simulink model "tests"  (R2024b)
settings: Solver=VariableStepAuto  StartTime=0.0  StopTime=1  RelTol=1e-3  AbsTol=1e-3  EnableMultiTasking=on
values from neighbouring files (symbols this model uses):
  m = obj.Br *obj.volume / obj.mu    [External_Magnet2.m]
  N = gridSizes(k)    [Test.m]
  Params = Sim_Param_Setup    [Sim_Open.m]
undefined symbols (not defined in the file or in its folder): X, Y, Z
libraries: sm_lib x88, vrlib x72, nesl_utility x52, matrix_library x46, sharedtransform x6
(part 3 of 5)

== system tests/Subsystem/Single_Arm/Plate_2/Torques and Forces ==
  m_slave : Inport
  Pos_Slave : Inport  Port=2
  M1 : Inport  Port=3
  Pos_Plate1 : Inport  Port=4
  M3 : Inport  Port=5
  Pos_Plate3 : Inport  Port=6
  M4 : Inport  Port=7
  Pos_Plate4 : Inport  Port=8
  M5 : Inport  Port=9
  Pos_Plate5 : Inport  Port=10
  M6 : Inport  Port=11
  Pos_Plate6 : Inport  Port=12
  Add{,1..4} (5 alike) : Sum  Inputs=+-
  Magnetic Forces : Subsystem
  Magnetic Torques : Subsystem
      settings: PortSchema="{\"entries\":[{\"content\":{\"sides\":[{\"content\":{\"connectorIds\":[\"In1\",\"In2\",\"In3\",\"In4\",\"In5\",\"In6\",\"In7\",\"In8\",\"In9\",\"In10\",\"In11\"]},\"type\":\"ConnectorPlacement.EquallySpacedRectSide\",\"uuid\":\"6f05c61b-28f4-4565-bbea-1be0fb93c6f0\"},{\"content\":{\"connectorIds\":[\"Out1\"],\"side\":\"RIGHT\"},\"type\":\"ConnectorPlacement.EquallySpacedRectSide\",\"uuid\":\"8634642c-fc93-4182-aaec-4f6aca47cd70\"},{\"content\":{\"connectorIds\":[\"LConn1\"],\"side\":\"TOP\"},\"type\":\"ConnectorPlacement.EquallySpacedRectSide\",\"uuid\":\"4c29c46f-a8de-4915-ac6e-9828579e7b84\"}]},\"type\":\"ConnectorPlacement.EquallySpacedConnector\",\"uuid\":\"3da81916-5d74-4352-a0fa-851a5433a86b\"}],\"packageUris\":[\"http://schema.mathworks.com/mf0/Connector/R2020b\"],\"version\":\"1.0\"}"
  brick reference : PMIOPort  Side=Left
  Forces : Outport
  Torques : Outport  Port=2
  wires:
  m_slave/1 -> Magnetic Forces/1(m_slave), Magnetic Torques/1(m_slave)
  Pos_Slave/1 -> Add4/1, Add3/1, Add2/1, Add1/1, Add/1
  Pos_Plate1/1 -> Add/2
  M1/1 -> Magnetic Torques/2(M1), Magnetic Forces/2(M1)
  Add/1 -> Magnetic Torques/7(r1), Magnetic Forces/7(r1)
  Pos_Plate6/1 -> Add4/2
  Pos_Plate5/1 -> Add3/2
  Pos_Plate4/1 -> Add2/2
  Pos_Plate3/1 -> Add1/2
  M3/1 -> Magnetic Forces/3(M3), Magnetic Torques/3(M3)
  Add1/1 -> Magnetic Torques/8(r3), Magnetic Forces/8(r3)
  M4/1 -> Magnetic Forces/4(M4), Magnetic Torques/4(M4)
  M5/1 -> Magnetic Forces/5(M5), Magnetic Torques/5(M5)
  M6/1 -> Magnetic Forces/6(M6), Magnetic Torques/6(M6)
  Add2/1 -> Magnetic Forces/9(r4), Magnetic Torques/9(r4)
  Add3/1 -> Magnetic Forces/10(r5), Magnetic Torques/10(r5)
  Add4/1 -> Magnetic Forces/11(r6), Magnetic Torques/11(r6)
  Magnetic Forces/1(Forces) -> Forces/1
  Magnetic Torques/1(Torque) -> Torques/1
  connections:
  brick reference/RConn1 -- Magnetic Torques/LConn1

== system tests/Subsystem/Single_Arm/Plate_3/Subsystem ==
  Slave_Moment : Inport
  Slave_Pos : Inport  Port=2
  Source_Moment : Inport  Port=3
  Source_Pos : Inport  Port=4
  Add : Sum  Inputs=+-
  Add1 : Sum  Inputs=+-
  Add2 : Sum  Inputs=+-
  Add3 : Sum  Inputs=+++
  Constant : Constant  Value=-3
  Constant1 : Constant  Value=-4
  Cross Product : matrix_library/Cross Product
  Dot Product : DotProduct  OutDataTypeStr=Inherit: Inherit via internal rule
  Dot Product1 : DotProduct  OutDataTypeStr=Inherit: Inherit via internal rule
  Gain : Gain  Gain=4*pi*1e-7/(4*pi)
  Gain1 : Gain  Gain=3
  Gain2 : Gain  Gain=3*4*pi*1e-7/(4*pi)
  Gain3 : Gain  Gain=5
  IdentityMatrix : IdentityMatrix  OutputDimensions=3
  Matrix Multiply : Product  Multiplication=Matrix(*)
  Matrix Multiply1 : Product  Multiplication=Matrix(*)
  Normalize Vector : vrlib/Utilities/Normalize Vector  maxzero=0
  Normalize Vector1 : vrlib/Utilities/Normalize Vector  maxzero=0
  Power : Math  Operator=pow
  Power1 : Math  Operator=pow
  Product{,1..5} (6 alike) : Product
  Sqrt : Sqrt
  Sqrt1 : Sqrt
  Transpose : Math  Operator=transpose
  m dot m : DotProduct  OutDataTypeStr=Inherit: Inherit via internal rule
  r dot m_master : DotProduct  OutDataTypeStr=Inherit: Inherit via internal rule
  r dot m_slave : DotProduct  OutDataTypeStr=Inherit: Inherit via internal rule
  Source_Torque : Outport
  Source_Force : Outport  Port=2
  wires:
  Power/1 -> Gain/1
  Transpose/1 -> Matrix Multiply/2
  Gain1/1 -> Add/1
  Matrix Multiply/1 -> Gain1/1
  Sqrt/1 -> Power/1
  Gain/1 -> Product/2
  Dot Product/1 -> Sqrt/1
  Product/1 -> Cross Product/2
  Matrix Multiply1/1 -> Product/1
  Normalize Vector/1 -> Transpose/1, Matrix Multiply/1
  IdentityMatrix/1 -> Add/2
  Constant/1 -> Power/2
  Add/1 -> Matrix Multiply1/1
  Slave_Pos/1 -> Add1/1
  Source_Pos/1 -> Add1/2
  Cross Product/1 -> Source_Torque/1
  Slave_Moment/1 -> Cross Product/1, Product2/2, m dot m/1, r dot m_slave/2
  Normalize Vector1/1 -> r dot m_slave/1, r dot m_master/1, Product4/2
  Add3/1 -> Product5/2
  Gain2/1 -> Product5/1
  Product4/1 -> Add3/3
  Dot Product1/1 -> Sqrt1/1
  Gain3/1 -> Add2/2
  r dot m_master/1 -> Product3/2, Product2/1
  Source_Moment/1 -> Matrix Multiply1/2, m dot m/2, Product1/2, r dot m_master/2
  m dot m/1 -> Add2/1
  Power1/1 -> Gain2/1
  Sqrt1/1 -> Power1/1
  r dot m_slave/1 -> Product1/1, Product3/1
  Product2/1 -> Add3/2
  Constant1/1 -> Power1/2
  Add2/1 -> Product4/1
  Add1/1 -> Normalize Vector1/1, Dot Product1/2, Dot Product1/1, Dot Product/2, Dot Product/1, Normalize Vector/1
  Product3/1 -> Gain3/1
  Product1/1 -> Add3/1
  Product5/1 -> Source_Force/1

== system tests/Subsystem/Single_Arm/Plate_3/Torques and Forces ==
  m_slave : Inport
  Pos_Slave : Inport  Port=2
  M1 : Inport  Port=3
  Pos_Plate1 : Inport  Port=4
  M2 : Inport  Port=5
  Pos_Plate2 : Inport  Port=6
  M4 : Inport  Port=7
  Pos_Plate4 : Inport  Port=8
  M5 : Inport  Port=9
  Pos_Plate5 : Inport  Port=10
  M6 : Inport  Port=11
  Pos_Plate6 : Inport  Port=12
  Add{,1..4} (5 alike) : Sum  Inputs=+-
  Magnetic Forces : Subsystem
  Magnetic Torques : Subsystem
      settings: PortSchema="{\"entries\":[{\"content\":{\"sides\":[{\"content\":{\"connectorIds\":[\"In1\",\"In2\",\"In3\",\"In4\",\"In5\",\"In6\",\"In7\",\"In8\",\"In9\",\"In10\",\"In11\"]},\"type\":\"ConnectorPlacement.EquallySpacedRectSide\",\"uuid\":\"05771496-45a2-4580-b6ab-cadf9064ee26\"},{\"content\":{\"connectorIds\":[\"Out1\"],\"side\":\"RIGHT\"},\"type\":\"ConnectorPlacement.EquallySpacedRectSide\",\"uuid\":\"b79900f2-9f02-4790-af3a-0fbba66daa11\"},{\"content\":{\"connectorIds\":[\"LConn1\"],\"side\":\"TOP\"},\"type\":\"ConnectorPlacement.EquallySpacedRectSide\",\"uuid\":\"95266051-22b3-46d7-add2-de0ce2a92008\"}]},\"type\":\"ConnectorPlacement.EquallySpacedConnector\",\"uuid\":\"2bf1b23d-6512-437d-b945-3c726b6a255c\"}],\"packageUris\":[\"http://schema.mathworks.com/mf0/Connector/R2020b\"],\"version\":\"1.0\"}"
  brick reference : PMIOPort  Side=Left
  Forces : Outport
  Torques : Outport  Port=2
  wires:
  m_slave/1 -> Magnetic Forces/1(m_slave), Magnetic Torques/1(m_slave)
  Pos_Slave/1 -> Add4/1, Add3/1, Add2/1, Add1/1, Add/1
  Pos_Plate1/1 -> Add/2
  M1/1 -> Magnetic Torques/2(M1), Magnetic Forces/2(M1)
  Add/1 -> Magnetic Torques/7(r1), Magnetic Forces/7(r1)
  Pos_Plate6/1 -> Add4/2
  Pos_Plate5/1 -> Add3/2
  Pos_Plate4/1 -> Add2/2
  Pos_Plate2/1 -> Add1/2
  M2/1 -> Magnetic Forces/3(M2), Magnetic Torques/3(M2)
  Add1/1 -> Magnetic Torques/8(r2), Magnetic Forces/8(r2)
  M4/1 -> Magnetic Forces/4(M4), Magnetic Torques/4(M4)
  M5/1 -> Magnetic Forces/5(M5), Magnetic Torques/5(M5)
  M6/1 -> Magnetic Forces/6(M6), Magnetic Torques/6(M6)
  Add2/1 -> Magnetic Forces/9(r4), Magnetic Torques/9(r4)
  Add3/1 -> Magnetic Forces/10(r5), Magnetic Torques/10(r5)
  Add4/1 -> Magnetic Forces/11(r6), Magnetic Torques/11(r6)
  Magnetic Forces/1(Forces) -> Forces/1
  Magnetic Torques/1(Torque) -> Torques/1
  connections:
  brick reference/RConn1 -- Magnetic Torques/LConn1

== system tests/Subsystem/Single_Arm/Plate_4/Subsystem ==
  Slave_Moment : Inport
  Slave_Pos : Inport  Port=2
  Source_Moment : Inport  Port=3
  Source_Pos : Inport  Port=4
  Add : Sum  Inputs=+-
  Add1 : Sum  Inputs=+-
  Add2 : Sum  Inputs=+-
  Add3 : Sum  Inputs=+++
  Constant : Constant  Value=-3
  Constant1 : Constant  Value=-4
  Cross Product : matrix_library/Cross Product
  Dot Product : DotProduct  OutDataTypeStr=Inherit: Inherit via internal rule
  Dot Product1 : DotProduct  OutDataTypeStr=Inherit: Inherit via internal rule
  Gain : Gain  Gain=4*pi*1e-7/(4*pi)
  Gain1 : Gain  Gain=3
  Gain2 : Gain  Gain=3*4*pi*1e-7/(4*pi)
  Gain3 : Gain  Gain=5
  IdentityMatrix : IdentityMatrix  OutputDimensions=3
  Matrix Multiply : Product  Multiplication=Matrix(*)
  Matrix Multiply1 : Product  Multiplication=Matrix(*)
  Normalize Vector : vrlib/Utilities/Normalize Vector  maxzero=0
  Normalize Vector1 : vrlib/Utilities/Normalize Vector  maxzero=0
  Power : Math  Operator=pow
  Power1 : Math  Operator=pow
  Product{,1..5} (6 alike) : Product
  Sqrt : Sqrt
  Sqrt1 : Sqrt
  Transpose : Math  Operator=transpose
  m dot m : DotProduct  OutDataTypeStr=Inherit: Inherit via internal rule
  r dot m_master : DotProduct  OutDataTypeStr=Inherit: Inherit via internal rule
  r dot m_slave : DotProduct  OutDataTypeStr=Inherit: Inherit via internal rule
  Source_Torque : Outport
  Source_Force : Outport  Port=2
  wires:
  Power/1 -> Gain/1
  Transpose/1 -> Matrix Multiply/2
  Gain1/1 -> Add/1
  Matrix Multiply/1 -> Gain1/1
  Sqrt/1 -> Power/1
  Gain/1 -> Product/2
  Dot Product/1 -> Sqrt/1
  Product/1 -> Cross Product/2
  Matrix Multiply1/1 -> Product/1
  Normalize Vector/1 -> Transpose/1, Matrix Multiply/1
  IdentityMatrix/1 -> Add/2
  Constant/1 -> Power/2
  Add/1 -> Matrix Multiply1/1
  Slave_Pos/1 -> Add1/1
  Source_Pos/1 -> Add1/2
  Cross Product/1 -> Source_Torque/1
  Slave_Moment/1 -> Cross Product/1, Product2/2, m dot m/1, r dot m_slave/2
  Normalize Vector1/1 -> r dot m_slave/1, r dot m_master/1, Product4/2
  Add3/1 -> Product5/2
  Gain2/1 -> Product5/1
  Product4/1 -> Add3/3
  Dot Product1/1 -> Sqrt1/1
  Gain3/1 -> Add2/2
  r dot m_master/1 -> Product3/2, Product2/1
  Source_Moment/1 -> Matrix Multiply1/2, m dot m/2, Product1/2, r dot m_master/2
  m dot m/1 -> Add2/1
  Power1/1 -> Gain2/1
  Sqrt1/1 -> Power1/1
  r dot m_slave/1 -> Product1/1, Product3/1
  Product2/1 -> Add3/2
  Constant1/1 -> Power1/2
  Add2/1 -> Product4/1
  Add1/1 -> Normalize Vector1/1, Dot Product1/2, Dot Product1/1, Dot Product/2, Dot Product/1, Normalize Vector/1
  Product3/1 -> Gain3/1
  Product1/1 -> Add3/1
  Product5/1 -> Source_Force/1

== system tests/Subsystem/Single_Arm/Plate_4/Torques and Forces ==
  m_slave : Inport
  Pos_Slave : Inport  Port=2
  M1 : Inport  Port=3
  Pos_Plate1 : Inport  Port=4
  M2 : Inport  Port=5
  Pos_Plate2 : Inport  Port=6
  M3 : Inport  Port=7
  Pos_Plate3 : Inport  Port=8
  M5 : Inport  Port=9
  Pos_Plate5 : Inport  Port=10
  M6 : Inport  Port=11
  Pos_Plate6 : Inport  Port=12
  Add{,1..4} (5 alike) : Sum  Inputs=+-
  Magnetic Forces : Subsystem
  Magnetic Torques : Subsystem
      settings: PortSchema="{\"entries\":[{\"content\":{\"sides\":[{\"content\":{\"connectorIds\":[\"In1\",\"In2\",\"In3\",\"In4\",\"In5\",\"In6\",\"In7\",\"In8\",\"In9\",\"In10\",\"In11\"]},\"type\":\"ConnectorPlacement.EquallySpacedRectSide\",\"uuid\":\"05771496-45a2-4580-b6ab-cadf9064ee26\"},{\"content\":{\"connectorIds\":[\"Out1\"],\"side\":\"RIGHT\"},\"type\":\"ConnectorPlacement.EquallySpacedRectSide\",\"uuid\":\"b79900f2-9f02-4790-af3a-0fbba66daa11\"},{\"content\":{\"connectorIds\":[\"LConn1\"],\"side\":\"TOP\"},\"type\":\"ConnectorPlacement.EquallySpacedRectSide\",\"uuid\":\"95266051-22b3-46d7-add2-de0ce2a92008\"}]},\"type\":\"ConnectorPlacement.EquallySpacedConnector\",\"uuid\":\"2bf1b23d-6512-437d-b945-3c726b6a255c\"}],\"packageUris\":[\"http://schema.mathworks.com/mf0/Connector/R2020b\"],\"version\":\"1.0\"}"
  brick reference : PMIOPort  Side=Left
  Forces : Outport
  Torques : Outport  Port=2
  wires:
  m_slave/1 -> Magnetic Forces/1(m_slave), Magnetic Torques/1(m_slave)
  Pos_Slave/1 -> Add4/1, Add3/1, Add2/1, Add1/1, Add/1
  Pos_Plate1/1 -> Add/2
  M1/1 -> Magnetic Torques/2(M1), Magnetic Forces/2(M1)
  Add/1 -> Magnetic Torques/7(r1), Magnetic Forces/7(r1)
  Pos_Plate6/1 -> Add4/2
  Pos_Plate5/1 -> Add3/2
  Pos_Plate3/1 -> Add2/2
  Pos_Plate2/1 -> Add1/2
  M2/1 -> Magnetic Forces/3(M2), Magnetic Torques/3(M2)
  Add1/1 -> Magnetic Torques/8(r2), Magnetic Forces/8(r2)
  M3/1 -> Magnetic Forces/4(M3), Magnetic Torques/4(M3)
  M5/1 -> Magnetic Forces/5(M5), Magnetic Torques/5(M5)
  M6/1 -> Magnetic Forces/6(M6), Magnetic Torques/6(M6)
  Add2/1 -> Magnetic Forces/9(r3), Magnetic Torques/9(r3)
  Add3/1 -> Magnetic Forces/10(r5), Magnetic Torques/10(r5)
  Add4/1 -> Magnetic Forces/11(r6), Magnetic Torques/11(r6)
  Magnetic Forces/1(Forces) -> Forces/1
  Magnetic Torques/1(Torque) -> Torques/1
  connections:
  brick reference/RConn1 -- Magnetic Torques/LConn1

== system tests/Subsystem/Single_Arm/Plate_5/Subsystem ==
  Slave_Moment : Inport
  Slave_Pos : Inport  Port=2
  Source_Moment : Inport  Port=3
  Source_Pos : Inport  Port=4
  Add : Sum  Inputs=+-
  Add1 : Sum  Inputs=+-
  Add2 : Sum  Inputs=+-
  Add3 : Sum  Inputs=+++
  Constant : Constant  Value=-3
  Constant1 : Constant  Value=-4
  Cross Product : matrix_library/Cross Product
  Dot Product : DotProduct  OutDataTypeStr=Inherit: Inherit via internal rule
  Dot Product1 : DotProduct  OutDataTypeStr=Inherit: Inherit via internal rule
  Gain : Gain  Gain=4*pi*1e-7/(4*pi)
  Gain1 : Gain  Gain=3
  Gain2 : Gain  Gain=3*4*pi*1e-7/(4*pi)
  Gain3 : Gain  Gain=5
  IdentityMatrix : IdentityMatrix  OutputDimensions=3
  Matrix Multiply : Product  Multiplication=Matrix(*)
  Matrix Multiply1 : Product  Multiplication=Matrix(*)
  Normalize Vector : vrlib/Utilities/Normalize Vector  maxzero=0
  Normalize Vector1 : vrlib/Utilities/Normalize Vector  maxzero=0
  Power : Math  Operator=pow
  Power1 : Math  Operator=pow
  Product{,1..5} (6 alike) : Product
  Sqrt : Sqrt
  Sqrt1 : Sqrt
  Transpose : Math  Operator=transpose
  m dot m : DotProduct  OutDataTypeStr=Inherit: Inherit via internal rule
  r dot m_master : DotProduct  OutDataTypeStr=Inherit: Inherit via internal rule
  r dot m_slave : DotProduct  OutDataTypeStr=Inherit: Inherit via internal rule
  Source_Torque : Outport
  Source_Force : Outport  Port=2
  wires:
  Power/1 -> Gain/1
  Transpose/1 -> Matrix Multiply/2
  Gain1/1 -> Add/1
  Matrix Multiply/1 -> Gain1/1
  Sqrt/1 -> Power/1
  Gain/1 -> Product/2
  Dot Product/1 -> Sqrt/1
  Product/1 -> Cross Product/2
  Matrix Multiply1/1 -> Product/1
  Normalize Vector/1 -> Transpose/1, Matrix Multiply/1
  IdentityMatrix/1 -> Add/2
  Constant/1 -> Power/2
  Add/1 -> Matrix Multiply1/1
  Slave_Pos/1 -> Add1/1
  Source_Pos/1 -> Add1/2
  Cross Product/1 -> Source_Torque/1
  Slave_Moment/1 -> Cross Product/1, Product2/2, m dot m/1, r dot m_slave/2
  Normalize Vector1/1 -> r dot m_slave/1, r dot m_master/1, Product4/2
  Add3/1 -> Product5/2
  Gain2/1 -> Product5/1
  Product4/1 -> Add3/3
  Dot Product1/1 -> Sqrt1/1
  Gain3/1 -> Add2/2
  r dot m_master/1 -> Product3/2, Product2/1
  Source_Moment/1 -> Matrix Multiply1/2, m dot m/2, Product1/2, r dot m_master/2
  m dot m/1 -> Add2/1
  Power1/1 -> Gain2/1
  Sqrt1/1 -> Power1/1
  r dot m_slave/1 -> Product1/1, Product3/1
  Product2/1 -> Add3/2
  Constant1/1 -> Power1/2
  Add2/1 -> Product4/1
  Add1/1 -> Normalize Vector1/1, Dot Product1/2, Dot Product1/1, Dot Product/2, Dot Product/1, Normalize Vector/1
  Product3/1 -> Gain3/1
  Product1/1 -> Add3/1
  Product5/1 -> Source_Force/1

== system tests/Subsystem/Single_Arm/Plate_5/Torques and Forces ==
  m_slave : Inport
  Pos_Slave : Inport  Port=2
  M1 : Inport  Port=3
  Pos_Plate1 : Inport  Port=4
  M2 : Inport  Port=5
  Pos_Plate2 : Inport  Port=6
  M3 : Inport  Port=7
  Pos_Plate3 : Inport  Port=8
  M4 : Inport  Port=9
  Pos_Plate4 : Inport  Port=10
  M6 : Inport  Port=11
  Pos_Plate6 : Inport  Port=12
  Add{,1..4} (5 alike) : Sum  Inputs=+-
  Magnetic Forces : Subsystem
  Magnetic Torques : Subsystem
      settings: PortSchema="{\"entries\":[{\"content\":{\"sides\":[{\"content\":{\"connectorIds\":[\"In1\",\"In2\",\"In3\",\"In4\",\"In5\",\"In6\",\"In7\",\"In8\",\"In9\",\"In10\",\"In11\"]},\"type\":\"ConnectorPlacement.EquallySpacedRectSide\",\"uuid\":\"05771496-45a2-4580-b6ab-cadf9064ee26\"},{\"content\":{\"connectorIds\":[\"Out1\"],\"side\":\"RIGHT\"},\"type\":\"ConnectorPlacement.EquallySpacedRectSide\",\"uuid\":\"b79900f2-9f02-4790-af3a-0fbba66daa11\"},{\"content\":{\"connectorIds\":[\"LConn1\"],\"side\":\"TOP\"},\"type\":\"ConnectorPlacement.EquallySpacedRectSide\",\"uuid\":\"95266051-22b3-46d7-add2-de0ce2a92008\"}]},\"type\":\"ConnectorPlacement.EquallySpacedConnector\",\"uuid\":\"2bf1b23d-6512-437d-b945-3c726b6a255c\"}],\"packageUris\":[\"http://schema.mathworks.com/mf0/Connector/R2020b\"],\"version\":\"1.0\"}"
  brick reference : PMIOPort  Side=Left
  Forces : Outport
  Torques : Outport  Port=2
  wires:
  m_slave/1 -> Magnetic Forces/1(m_slave), Magnetic Torques/1(m_slave)
  Pos_Slave/1 -> Add4/1, Add3/1, Add2/1, Add1/1, Add/1
  Pos_Plate1/1 -> Add/2
  M1/1 -> Magnetic Torques/2(M1), Magnetic Forces/2(M1)
  Add/1 -> Magnetic Torques/7(r1), Magnetic Forces/7(r1)
  Pos_Plate6/1 -> Add4/2
  Pos_Plate4/1 -> Add3/2
  Pos_Plate3/1 -> Add2/2
  Pos_Plate2/1 -> Add1/2
  M2/1 -> Magnetic Forces/3(M2), Magnetic Torques/3(M2)
  Add1/1 -> Magnetic Torques/8(r2), Magnetic Forces/8(r2)
  M3/1 -> Magnetic Forces/4(M3), Magnetic Torques/4(M3)
  M4/1 -> Magnetic Forces/5(M4), Magnetic Torques/5(M4)
  M6/1 -> Magnetic Forces/6(M6), Magnetic Torques/6(M6)
  Add2/1 -> Magnetic Forces/9(r3), Magnetic Torques/9(r3)
  Add3/1 -> Magnetic Forces/10(r4), Magnetic Torques/10(r4)
  Add4/1 -> Magnetic Forces/11(r6), Magnetic Torques/11(r6)
  Magnetic Forces/1(Forces) -> Forces/1
  Magnetic Torques/1(Torque) -> Torques/1
  connections:
  brick reference/RConn1 -- Magnetic Torques/LConn1

== system tests/Subsystem/Single_Arm/Plate_6/Subsystem ==
  Slave_Moment : Inport
  Slave_Pos : Inport  Port=2
  Source_Moment : Inport  Port=3
  Source_Pos : Inport  Port=4
  Add : Sum  Inputs=+-
  Add1 : Sum  Inputs=+-
  Add2 : Sum  Inputs=+-
  Add3 : Sum  Inputs=+++
  Constant : Constant  Value=-3
  Constant1 : Constant  Value=-4
  Cross Product : matrix_library/Cross Product
  Dot Product : DotProduct  OutDataTypeStr=Inherit: Inherit via internal rule
  Dot Product1 : DotProduct  OutDataTypeStr=Inherit: Inherit via internal rule
  Gain : Gain  Gain=4*pi*1e-7/(4*pi)
  Gain1 : Gain  Gain=3
  Gain2 : Gain  Gain=3*4*pi*1e-7/(4*pi)
  Gain3 : Gain  Gain=5
  IdentityMatrix : IdentityMatrix  OutputDimensions=3
  Matrix Multiply : Product  Multiplication=Matrix(*)
  Matrix Multiply1 : Product  Multiplication=Matrix(*)
  Normalize Vector : vrlib/Utilities/Normalize Vector  maxzero=0
  Normalize Vector1 : vrlib/Utilities/Normalize Vector  maxzero=0
  Power : Math  Operator=pow
  Power1 : Math  Operator=pow
  Product{,1..5} (6 alike) : Product
  Sqrt : Sqrt
  Sqrt1 : Sqrt
  Transpose : Math  Operator=transpose
  m dot m : DotProduct  OutDataTypeStr=Inherit: Inherit via internal rule
  r dot m_master : DotProduct  OutDataTypeStr=Inherit: Inherit via internal rule
  r dot m_slave : DotProduct  OutDataTypeStr=Inherit: Inherit via internal rule
  Source_Torque : Outport
  Source_Force : Outport  Port=2
  wires:
  Power/1 -> Gain/1
  Transpose/1 -> Matrix Multiply/2
  Gain1/1 -> Add/1
  Matrix Multiply/1 -> Gain1/1
  Sqrt/1 -> Power/1
  Gain/1 -> Product/2
  Dot Product/1 -> Sqrt/1
  Product/1 -> Cross Product/2
  Matrix Multiply1/1 -> Product/1
  Normalize Vector/1 -> Transpose/1, Matrix Multiply/1
  IdentityMatrix/1 -> Add/2
  Constant/1 -> Power/2
  Add/1 -> Matrix Multiply1/1
  Slave_Pos/1 -> Add1/1
  Source_Pos/1 -> Add1/2
  Cross Product/1 -> Source_Torque/1
  Slave_Moment/1 -> Cross Product/1, Product2/2, m dot m/1, r dot m_slave/2
  Normalize Vector1/1 -> r dot m_slave/1, r dot m_master/1, Product4/2
  Add3/1 -> Product5/2
  Gain2/1 -> Product5/1
  Product4/1 -> Add3/3
  Dot Product1/1 -> Sqrt1/1
  Gain3/1 -> Add2/2
  r dot m_master/1 -> Product3/2, Product2/1
  Source_Moment/1 -> Matrix Multiply1/2, m dot m/2, Product1/2, r dot m_master/2
  m dot m/1 -> Add2/1
  Power1/1 -> Gain2/1
  Sqrt1/1 -> Power1/1
  r dot m_slave/1 -> Product1/1, Product3/1
  Product2/1 -> Add3/2
  Constant1/1 -> Power1/2
  Add2/1 -> Product4/1
  Add1/1 -> Normalize Vector1/1, Dot Product1/2, Dot Product1/1, Dot Product/2, Dot Product/1, Normalize Vector/1
  Product3/1 -> Gain3/1
  Product1/1 -> Add3/1
  Product5/1 -> Source_Force/1

== system tests/Subsystem/Single_Arm/Plate_6/Torques and Forces ==
  m_slave : Inport
  Pos_Slave : Inport  Port=2
  M1 : Inport  Port=3
  Pos_Plate1 : Inport  Port=4
  M2 : Inport  Port=5
  Pos_Plate2 : Inport  Port=6
  M3 : Inport  Port=7
  Pos_Plate3 : Inport  Port=8
  M4 : Inport  Port=9
  Pos_Plate4 : Inport  Port=10
  M5 : Inport  Port=11
  Pos_Plate5 : Inport  Port=12
  Add{,1..4} (5 alike) : Sum  Inputs=+-
  Magnetic Forces : Subsystem
  Magnetic Torques : Subsystem
      settings: PortSchema="{\"entries\":[{\"content\":{\"sides\":[{\"content\":{\"connectorIds\":[\"In1\",\"In2\",\"In3\",\"In4\",\"In5\",\"In6\",\"In7\",\"In8\",\"In9\",\"In10\",\"In11\"]},\"type\":\"ConnectorPlacement.EquallySpacedRectSide\",\"uuid\":\"6f05c61b-28f4-4565-bbea-1be0fb93c6f0\"},{\"content\":{\"connectorIds\":[\"Out1\"],\"side\":\"RIGHT\"},\"type\":\"ConnectorPlacement.EquallySpacedRectSide\",\"uuid\":\"8634642c-fc93-4182-aaec-4f6aca47cd70\"},{\"content\":{\"connectorIds\":[\"LConn1\"],\"side\":\"TOP\"},\"type\":\"ConnectorPlacement.EquallySpacedRectSide\",\"uuid\":\"4c29c46f-a8de-4915-ac6e-9828579e7b84\"}]},\"type\":\"ConnectorPlacement.EquallySpacedConnector\",\"uuid\":\"3da81916-5d74-4352-a0fa-851a5433a86b\"}],\"packageUris\":[\"http://schema.mathworks.com/mf0/Connector/R2020b\"],\"version\":\"1.0\"}"
  Brick reference : PMIOPort  Side=Left
  Forces : Outport
  Torques : Outport  Port=2
  wires:
  m_slave/1 -> Magnetic Forces/1(m_slave), Magnetic Torques/1(m_slave)
  Pos_Slave/1 -> Add4/1, Add3/1, Add2/1, Add1/1, Add/1
  Pos_Plate1/1 -> Add/2
  M1/1 -> Magnetic Torques/2(M1), Magnetic Forces/2(M1)
  Add/1 -> Magnetic Torques/7(r1), Magnetic Forces/7(r1)
  Pos_Plate5/1 -> Add4/2
  Pos_Plate4/1 -> Add3/2
  Pos_Plate3/1 -> Add2/2
  Pos_Plate2/1 -> Add1/2
  M2/1 -> Magnetic Forces/3(M2), Magnetic Torques/3(M2)
  Add1/1 -> Magnetic Torques/8(r2), Magnetic Forces/8(r2)
  M3/1 -> Magnetic Forces/4(M3), Magnetic Torques/4(M3)
  M4/1 -> Magnetic Forces/5(M4), Magnetic Torques/5(M4)
  M5/1 -> Magnetic Forces/6(M5), Magnetic Torques/6(M5)
  Add2/1 -> Magnetic Forces/9(r3), Magnetic Torques/9(r3)
  Add3/1 -> Magnetic Forces/10(r4), Magnetic Torques/10(r4)
  Add4/1 -> Magnetic Forces/11(r5), Magnetic Torques/11(r5)
  Magnetic Forces/1(Forces) -> Forces/1
  Magnetic Torques/1(Torque) -> Torques/1
  connections:
  Brick reference/RConn1 -- Magnetic Torques/LConn1

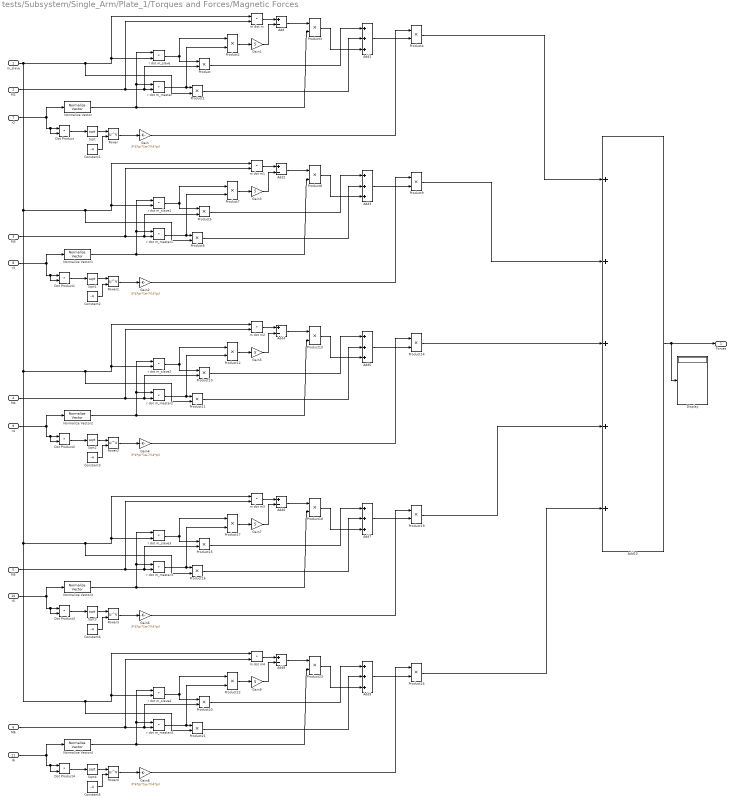
== system tests/Subsystem/Single_Arm/Plate_1/Torques and Forces/Magnetic Forces ==
  m_slave : Inport
  M2 : Inport  Port=2
  M3 : Inport  Port=3
  M4 : Inport  Port=4
  M5 : Inport  Port=5
  M6 : Inport  Port=6
  r2 : Inport  Port=7
  r3 : Inport  Port=8
  r4 : Inport  Port=9
  r5 : Inport  Port=10
  r6 : Inport  Port=11
  Add{,2,4,6,8} (5 alike) : Sum  Inputs=+-
  Add{1,3,5,7,9} (5 alike) : Sum  Inputs=+++
  Add10 : Sum  Inputs=+++++
  Constant{1..5} (5 alike) : Constant  Value=-4
  Display : Display
  Dot Product{,1..4} (5 alike) : DotProduct  OutDataTypeStr=Inherit: Inherit via internal rule
  Gain{,2,4,6,8} (5 alike) : Gain  Gain=3*4*pi*1e-7/(4*pi)
  Gain{1,3,5,7,9} (5 alike) : Gain  Gain=5
  Normalize Vector{,1..4} (5 alike) : vrlib/Utilities/Normalize Vector  maxzero=0
  Power{,1..4} (5 alike) : Math  Operator=pow
  Product{,1..24} (25 alike) : Product
  Sqrt{,1..4} (5 alike) : Sqrt
  m dot m{,1..4} (5 alike) : DotProduct  OutDataTypeStr=Inherit: Inherit via internal rule
  r dot m_master{,1..4} (5 alike) : DotProduct  OutDataTypeStr=Inherit: Inherit via internal rule
  r dot m_slave{,1..4} (5 alike) : DotProduct  OutDataTypeStr=Inherit: Inherit via internal rule
  Forces : Outport
  wires:
  M2/1 -> m dot m/2, Product/2, r dot m_master/2
  r2/1 -> Normalize Vector/1, Dot Product/2, Dot Product/1
  Dot Product/1 -> Sqrt/1
  Sqrt/1 -> Power/1
  Constant1/1 -> Power/2
  Power/1 -> Gain/1
  r dot m_slave/1 -> Product/1, Product2/1
  r dot m_master/1 -> Product2/2, Product1/1
  Product/1 -> Add1/1
  Product1/1 -> Add1/2
  Product2/1 -> Gain1/1
  m dot m/1 -> Add/1
  Gain1/1 -> Add/2
  Normalize Vector/1 -> r dot m_slave/1, r dot m_master/1, Product3/2
  Add/1 -> Product3/1
  Product3/1 -> Add1/3
  Gain/1 -> Product4/1
  Add1/1 -> Product4/2
  Dot Product1/1 -> Sqrt1/1
  Normalize Vector1/1 -> r dot m_slave1/1, r dot m_master1/1, Product8/2
  Product5/1 -> Add3/1
  Add2/1 -> Product8/1
  Gain3/1 -> Add2/2
  m dot m1/1 -> Add2/1
  r dot m_master1/1 -> Product7/2, Product6/1
  Gain2/1 -> Product9/1
  Power1/1 -> Gain2/1
  M3/1 -> m dot m1/2, Product5/2, r dot m_master1/2
  Add3/1 -> Product9/2
  r3/1 -> Dot Product1/2, Dot Product1/1, Normalize Vector1/1
  Sqrt1/1 -> Power1/1
  Product9/1 -> Add10/2
  Product7/1 -> Gain3/1
  Constant2/1 -> Power1/2
  Product8/1 -> Add3/3
  Product6/1 -> Add3/2
  r dot m_slave1/1 -> Product5/1, Product7/1
  Dot Product2/1 -> Sqrt2/1
  Normalize Vector2/1 -> r dot m_slave2/1, r dot m_master2/1, Product13/2
  Product10/1 -> Add5/1
  Add4/1 -> Product13/1
  Gain5/1 -> Add4/2
  m dot m2/1 -> Add4/1
  r dot m_master2/1 -> Product12/2, Product11/1
  Gain4/1 -> Product14/1
  Power2/1 -> Gain4/1
  M4/1 -> m dot m2/2, Product10/2, r dot m_master2/2
  Add5/1 -> Product14/2
  r4/1 -> Normalize Vector2/1, Dot Product2/2, Dot Product2/1
  Sqrt2/1 -> Power2/1
  Product14/1 -> Add10/3
  Product12/1 -> Gain5/1
  Constant3/1 -> Power2/2
  Product13/1 -> Add5/3
  Product11/1 -> Add5/2
  r dot m_slave2/1 -> Product10/1, Product12/1
  Dot Product3/1 -> Sqrt3/1
  Normalize Vector3/1 -> r dot m_slave3/1, r dot m_master3/1, Product18/2
  Product15/1 -> Add7/1
  Add6/1 -> Product18/1
  Gain7/1 -> Add6/2
  m dot m3/1 -> Add6/1
  r dot m_master3/1 -> Product17/2, Product16/1
  Gain6/1 -> Product19/1
  Power3/1 -> Gain6/1
  M5/1 -> m dot m3/2, Product15/2, r dot m_master3/2
  Add7/1 -> Product19/2
  r5/1 -> Dot Product3/2, Dot Product3/1, Normalize Vector3/1
  Sqrt3/1 -> Power3/1
  Product19/1 -> Add10/4
  Product17/1 -> Gain7/1
  Constant4/1 -> Power3/2
  Product18/1 -> Add7/3
  Product16/1 -> Add7/2
  r dot m_slave3/1 -> Product15/1, Product17/1
  Dot Product4/1 -> Sqrt4/1
  Normalize Vector4/1 -> r dot m_slave4/1, r dot m_master4/1, Product23/2
  Product20/1 -> Add9/1
  Add8/1 -> Product23/1
  Gain9/1 -> Add8/2
  m dot m4/1 -> Add8/1
  r dot m_master4/1 -> Product22/2, Product21/1
  Gain8/1 -> Product24/1
  Power4/1 -> Gain8/1
  M6/1 -> m dot m4/2, Product20/2, r dot m_master4/2
  Add9/1 -> Product24/2
  r6/1 -> Normalize Vector4/1, Dot Product4/2, Dot Product4/1
  Sqrt4/1 -> Power4/1
  Product24/1 -> Add10/5
  Product22/1 -> Gain9/1
  Constant5/1 -> Power4/2
  m_slave/1 -> Product21/2, m dot m4/1, r dot m_slave4/2, Product16/2, m dot m3/1, r dot m_slave3/2, Product11/2, m dot m2/1, r dot m_slave2/2, Product6/2, m dot m1/1, r dot m_slave1/2, Product1/2, m dot m/1, r dot m_slave/2
  Product23/1 -> Add9/3
  Product21/1 -> Add9/2
  r dot m_slave4/1 -> Product20/1, Product22/1
  Product4/1 -> Add10/1
  Add10/1 -> Forces/1, Display/1

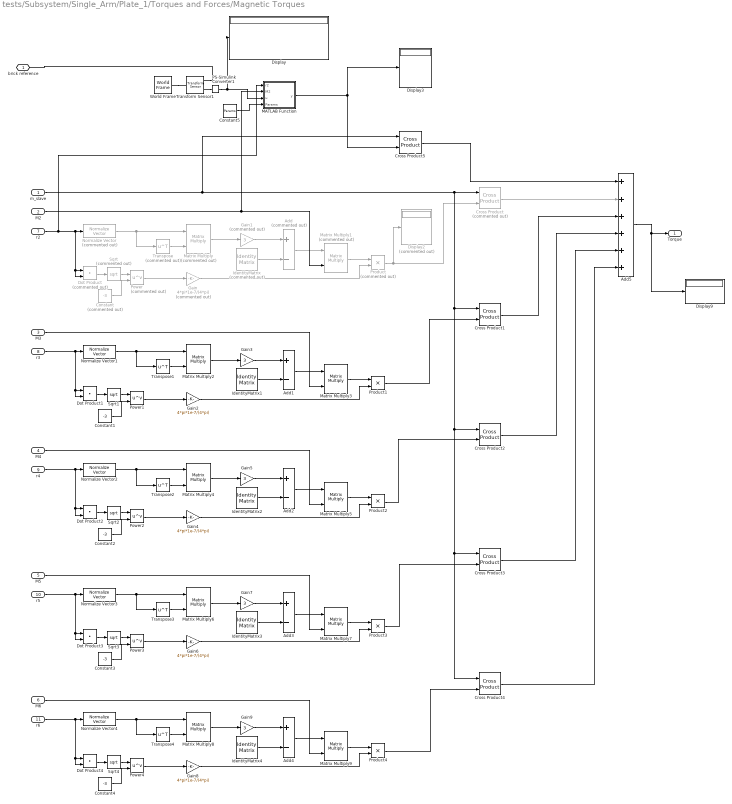
== system tests/Subsystem/Single_Arm/Plate_1/Torques and Forces/Magnetic Torques ==
  m_slave : Inport
  M2 : Inport  Port=2
  M3 : Inport  Port=3
  M4 : Inport  Port=4
  M5 : Inport  Port=5
  M6 : Inport  Port=6
  r2 : Inport  Port=7
  r3 : Inport  Port=8
  r4 : Inport  Port=9
  r5 : Inport  Port=10
  r6 : Inport  Port=11
  Add : Sum  Commented=on  Inputs=+-
  Add{1..4} (4 alike) : Sum  Inputs=+-
  Add5 : Sum  Inputs=++++++
  Constant : Constant  Commented=on  Value=-3
  Constant{1..4} (4 alike) : Constant  Value=-3
  Constant5 : Constant  Value=Params  OutDataTypeStr=Bus:slBus1
  Cross Product : matrix_library/Cross Product  Commented=on
  Cross Product{1..5} (5 alike) : matrix_library/Cross Product
  Display : Display
  Display2 : Display  Commented=on
  Display3 : Display
  Display9 : Display
  Dot Product : DotProduct  Commented=on  OutDataTypeStr=Inherit: Inherit via internal rule
  Dot Product{1..4} (4 alike) : DotProduct  OutDataTypeStr=Inherit: Inherit via internal rule
  Gain : Gain  Commented=on  Gain=4*pi*1e-7/(4*pi)
  Gain1 : Gain  Commented=on  Gain=3
  Gain{2,4,6,8} (4 alike) : Gain  Gain=4*pi*1e-7/(4*pi)
  Gain{3,5,7,9} (4 alike) : Gain  Gain=3
  IdentityMatrix : IdentityMatrix  Commented=on  OutputDimensions=3
  IdentityMatrix{1..4} (4 alike) : IdentityMatrix  OutputDimensions=3
  MATLAB Function : MATLAB Function  TreatAsAtomicUnit=on
  Matrix Multiply : Product  Commented=on  Multiplication=Matrix(*)
  Matrix Multiply1 : Product  Commented=on  Multiplication=Matrix(*)
  Matrix Multiply{2..9} (8 alike) : Product  Multiplication=Matrix(*)
  Normalize Vector : vrlib/Utilities/Normalize Vector  Commented=on  maxzero=0
  Normalize Vector{1..4} (4 alike) : vrlib/Utilities/Normalize Vector  maxzero=0
  PS-Simulink Converter1 : nesl_utility/PS-Simulink Converter  PhysicalDomain=network_engine_domain  SubClassName=ps_output  LeftPortType=input  RightPortType=output  PseudoPeriodic=off  Frequencies=[]  VectorFormat=inherit  Unit=inherit  AffineConversion=off
  Power : Math  Commented=on  Operator=pow
  Power{1..4} (4 alike) : Math  Operator=pow
  Product : Product  Commented=on
  Product{1..4} (4 alike) : Product
  Sqrt : Sqrt  Commented=on
  Sqrt{1..4} (4 alike) : Sqrt
  Transform Sensor1 : sm_lib/Frames and Transforms/Transform Sensor  MeasurementFrame=World  RotationSequence=XYX  SenseAngle=off  SenseAxis=off  SenseQ=off  SenseR=on  SenseRotationSequence=off  SenseOmegaX=off  SenseOmegaY=off  SenseOmegaZ=off  SenseOmega=off  SenseQDot=off  SenseRDot=off  SenseRotationSequenceDot=off  SenseAlphaX=off  SenseAlphaY=off  SenseAlphaZ=off  SenseAlpha=off  SenseQDDot=off  SenseRDDot=off  SenseX=off  SenseY=off  SenseZ=off  SenseXYZ=off  SenseRad=off  SenseAzim=off  SenseDist=off  SenseInc=off  SenseXDot=off  SenseYDot=off  SenseZDot=off  SenseXYZDot=off  SenseRadDot=off  SenseAzimDot=off  SenseDistDot=off  SenseIncDot=off  SenseXDDot=off  SenseYDDot=off  SenseZDDot=off  SenseXYZDDot=off  SenseRadDDot=off  SenseAzimDDot=off  SenseDistDDot=off  SenseIncDDot=off
  Transpose : Math  Commented=on  Operator=transpose
  Transpose{1..4} (4 alike) : Math  Operator=transpose
  World Frame : sm_lib/Frames and Transforms/World Frame
  brick reference : PMIOPort  Side=Left
  Torque : Outport
  wires:
  r2/1 -> MATLAB Function/1(r2), Dot Product/2, Dot Product/1, Normalize Vector/1
  Constant/1 -> Power/2
  Power/1 -> Gain/1
  Normalize Vector/1 -> Transpose/1, Matrix Multiply/1
  Transpose/1 -> Matrix Multiply/2
  Matrix Multiply/1 -> Gain1/1
  IdentityMatrix/1 -> Add/2
  Gain1/1 -> Add/1
  Add/1 -> Matrix Multiply1/1
  M2/1 -> MATLAB Function/2(M2), Matrix Multiply1/2
  Matrix Multiply1/1 -> Product/1
  Gain/1 -> Product/2
  Product/1 -> Cross Product/2, Display2/1
  m_slave/1 -> Cross Product5/1, Cross Product4/1, Cross Product3/1, Cross Product2/1, Cross Product1/1, Cross Product/1
  Dot Product/1 -> Sqrt/1
  Sqrt/1 -> Power/1
  Transpose1/1 -> Matrix Multiply2/2
  Normalize Vector1/1 -> Transpose1/1, Matrix Multiply2/1
  r3/1 -> Dot Product1/2, Dot Product1/1, Normalize Vector1/1
  Matrix Multiply3/1 -> Product1/1
  Matrix Multiply2/1 -> Gain3/1
  IdentityMatrix1/1 -> Add1/2
  Power1/1 -> Gain2/1
  M3/1 -> Matrix Multiply3/2
  Gain3/1 -> Add1/1
  Sqrt1/1 -> Power1/1
  Product1/1 -> Cross Product1/2
  Gain2/1 -> Product1/2
  Add1/1 -> Matrix Multiply3/1
  Dot Product1/1 -> Sqrt1/1
  Constant1/1 -> Power1/2
  Transpose2/1 -> Matrix Multiply4/2
  Normalize Vector2/1 -> Transpose2/1, Matrix Multiply4/1
  r4/1 -> Dot Product2/2, Dot Product2/1, Normalize Vector2/1
  Matrix Multiply5/1 -> Product2/1
  Matrix Multiply4/1 -> Gain5/1
  IdentityMatrix2/1 -> Add2/2
  Power2/1 -> Gain4/1
  M4/1 -> Matrix Multiply5/2
  Gain5/1 -> Add2/1
  Sqrt2/1 -> Power2/1
  Product2/1 -> Cross Product2/2
  Gain4/1 -> Product2/2
  Add2/1 -> Matrix Multiply5/1
  Dot Product2/1 -> Sqrt2/1
  Constant2/1 -> Power2/2
  Transpose3/1 -> Matrix Multiply6/2
  Normalize Vector3/1 -> Transpose3/1, Matrix Multiply6/1
  r5/1 -> Dot Product3/2, Dot Product3/1, Normalize Vector3/1
  Matrix Multiply7/1 -> Product3/1
  Matrix Multiply6/1 -> Gain7/1
  IdentityMatrix3/1 -> Add3/2
  Power3/1 -> Gain6/1
  M5/1 -> Matrix Multiply7/2
  Gain7/1 -> Add3/1
  Sqrt3/1 -> Power3/1
  Product3/1 -> Cross Product3/2
  Gain6/1 -> Product3/2
  Add3/1 -> Matrix Multiply7/1
  Dot Product3/1 -> Sqrt3/1
  Constant3/1 -> Power3/2
  Transpose4/1 -> Matrix Multiply8/2
  Normalize Vector4/1 -> Transpose4/1, Matrix Multiply8/1
  r6/1 -> Dot Product4/2, Dot Product4/1, Normalize Vector4/1
  Matrix Multiply9/1 -> Product4/1
  Matrix Multiply8/1 -> Gain9/1
  IdentityMatrix4/1 -> Add4/2
  Power4/1 -> Gain8/1
  M6/1 -> Matrix Multiply9/2
  Gain9/1 -> Add4/1
  Sqrt4/1 -> Power4/1
  Product4/1 -> Cross Product4/2
  Gain8/1 -> Product4/2
  Add4/1 -> Matrix Multiply9/1
  Dot Product4/1 -> Sqrt4/1
  Constant4/1 -> Power4/2
  Cross Product/1 -> Add5/2
  Cross Product1/1 -> Add5/3
  Cross Product2/1 -> Add5/4
  Cross Product3/1 -> Add5/5
  Cross Product4/1 -> Add5/6
  Add5/1 -> Display9/1, Torque/1
  Constant5/1 -> MATLAB Function/4(Params)
  PS-Simulink Converter1/1 -> Display/1, MATLAB Function/3(u)
  MATLAB Function/1(y) -> Cross Product5/2, Display3/1
  Cross Product5/1 -> Add5/1
  connections:
  Transform Sensor1/RConn1 -- brick reference/RConn1
  Transform Sensor1/RConn2 -- PS-Simulink Converter1/LConn1
  World Frame/RConn1 -- Transform Sensor1/LConn1

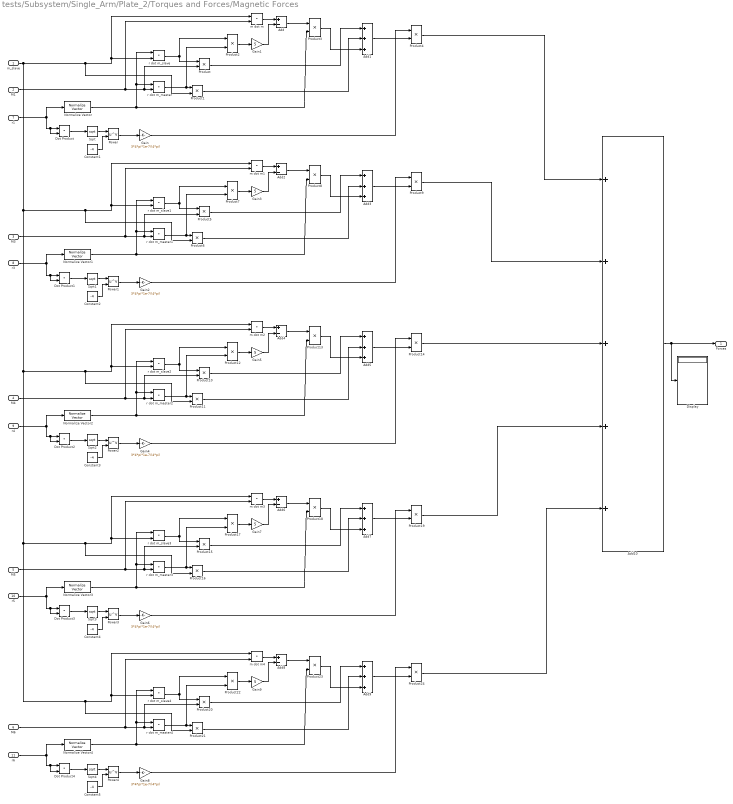
== system tests/Subsystem/Single_Arm/Plate_2/Torques and Forces/Magnetic Forces ==
  m_slave : Inport
  M1 : Inport  Port=2
  M3 : Inport  Port=3
  M4 : Inport  Port=4
  M5 : Inport  Port=5
  M6 : Inport  Port=6
  r1 : Inport  Port=7
  r3 : Inport  Port=8
  r4 : Inport  Port=9
  r5 : Inport  Port=10
  r6 : Inport  Port=11
  Add{,2,4,6,8} (5 alike) : Sum  Inputs=+-
  Add{1,3,5,7,9} (5 alike) : Sum  Inputs=+++
  Add10 : Sum  Inputs=+++++
  Constant{1..5} (5 alike) : Constant  Value=-4
  Display : Display
  Dot Product{,1..4} (5 alike) : DotProduct  OutDataTypeStr=Inherit: Inherit via internal rule
  Gain{,2,4,6,8} (5 alike) : Gain  Gain=3*4*pi*1e-7/(4*pi)
  Gain{1,3,5,7,9} (5 alike) : Gain  Gain=5
  Normalize Vector{,1..4} (5 alike) : vrlib/Utilities/Normalize Vector  maxzero=0
  Power{,1..4} (5 alike) : Math  Operator=pow
  Product{,1..24} (25 alike) : Product
  Sqrt{,1..4} (5 alike) : Sqrt
  m dot m{,1..4} (5 alike) : DotProduct  OutDataTypeStr=Inherit: Inherit via internal rule
  r dot m_master{,1..4} (5 alike) : DotProduct  OutDataTypeStr=Inherit: Inherit via internal rule
  r dot m_slave{,1..4} (5 alike) : DotProduct  OutDataTypeStr=Inherit: Inherit via internal rule
  Forces : Outport
  wires:
  M1/1 -> m dot m/2, Product/2, r dot m_master/2
  r1/1 -> Normalize Vector/1, Dot Product/2, Dot Product/1
  Dot Product/1 -> Sqrt/1
  Sqrt/1 -> Power/1
  Constant1/1 -> Power/2
  Power/1 -> Gain/1
  r dot m_slave/1 -> Product/1, Product2/1
  r dot m_master/1 -> Product2/2, Product1/1
  Product/1 -> Add1/1
  Product1/1 -> Add1/2
  Product2/1 -> Gain1/1
  m dot m/1 -> Add/1
  Gain1/1 -> Add/2
  Normalize Vector/1 -> r dot m_slave/1, r dot m_master/1, Product3/2
  Add/1 -> Product3/1
  Product3/1 -> Add1/3
  Gain/1 -> Product4/1
  Add1/1 -> Product4/2
  Dot Product1/1 -> Sqrt1/1
  Normalize Vector1/1 -> r dot m_slave1/1, r dot m_master1/1, Product8/2
  Product5/1 -> Add3/1
  Add2/1 -> Product8/1
  Gain3/1 -> Add2/2
  m dot m1/1 -> Add2/1
  r dot m_master1/1 -> Product7/2, Product6/1
  Gain2/1 -> Product9/1
  Power1/1 -> Gain2/1
  M3/1 -> m dot m1/2, Product5/2, r dot m_master1/2
  Add3/1 -> Product9/2
  r3/1 -> Dot Product1/2, Dot Product1/1, Normalize Vector1/1
  Sqrt1/1 -> Power1/1
  Product9/1 -> Add10/2
  Product7/1 -> Gain3/1
  Constant2/1 -> Power1/2
  Product8/1 -> Add3/3
  Product6/1 -> Add3/2
  r dot m_slave1/1 -> Product5/1, Product7/1
  Dot Product2/1 -> Sqrt2/1
  Normalize Vector2/1 -> r dot m_slave2/1, r dot m_master2/1, Product13/2
  Product10/1 -> Add5/1
  Add4/1 -> Product13/1
  Gain5/1 -> Add4/2
  m dot m2/1 -> Add4/1
  r dot m_master2/1 -> Product12/2, Product11/1
  Gain4/1 -> Product14/1
  Power2/1 -> Gain4/1
  M4/1 -> m dot m2/2, Product10/2, r dot m_master2/2
  Add5/1 -> Product14/2
  r4/1 -> Normalize Vector2/1, Dot Product2/2, Dot Product2/1
  Sqrt2/1 -> Power2/1
  Product14/1 -> Add10/3
  Product12/1 -> Gain5/1
  Constant3/1 -> Power2/2
  Product13/1 -> Add5/3
  Product11/1 -> Add5/2
  r dot m_slave2/1 -> Product10/1, Product12/1
  Dot Product3/1 -> Sqrt3/1
  Normalize Vector3/1 -> r dot m_slave3/1, r dot m_master3/1, Product18/2
  Product15/1 -> Add7/1
  Add6/1 -> Product18/1
  Gain7/1 -> Add6/2
  m dot m3/1 -> Add6/1
  r dot m_master3/1 -> Product17/2, Product16/1
  Gain6/1 -> Product19/1
  Power3/1 -> Gain6/1
  M5/1 -> m dot m3/2, Product15/2, r dot m_master3/2
  Add7/1 -> Product19/2
  r5/1 -> Dot Product3/2, Dot Product3/1, Normalize Vector3/1
  Sqrt3/1 -> Power3/1
  Product19/1 -> Add10/4
  Product17/1 -> Gain7/1
  Constant4/1 -> Power3/2
  Product18/1 -> Add7/3
  Product16/1 -> Add7/2
  r dot m_slave3/1 -> Product15/1, Product17/1
  Dot Product4/1 -> Sqrt4/1
  Normalize Vector4/1 -> r dot m_slave4/1, r dot m_master4/1, Product23/2
  Product20/1 -> Add9/1
  Add8/1 -> Product23/1
  Gain9/1 -> Add8/2
  m dot m4/1 -> Add8/1
  r dot m_master4/1 -> Product22/2, Product21/1
  Gain8/1 -> Product24/1
  Power4/1 -> Gain8/1
  M6/1 -> m dot m4/2, Product20/2, r dot m_master4/2
  Add9/1 -> Product24/2
  r6/1 -> Normalize Vector4/1, Dot Product4/2, Dot Product4/1
  Sqrt4/1 -> Power4/1
  Product24/1 -> Add10/5
  Product22/1 -> Gain9/1
  Constant5/1 -> Power4/2
  m_slave/1 -> Product21/2, m dot m4/1, r dot m_slave4/2, Product16/2, m dot m3/1, r dot m_slave3/2, Product11/2, m dot m2/1, r dot m_slave2/2, Product6/2, m dot m1/1, r dot m_slave1/2, Product1/2, m dot m/1, r dot m_slave/2
  Product23/1 -> Add9/3
  Product21/1 -> Add9/2
  r dot m_slave4/1 -> Product20/1, Product22/1
  Product4/1 -> Add10/1
  Add10/1 -> Forces/1, Display/1

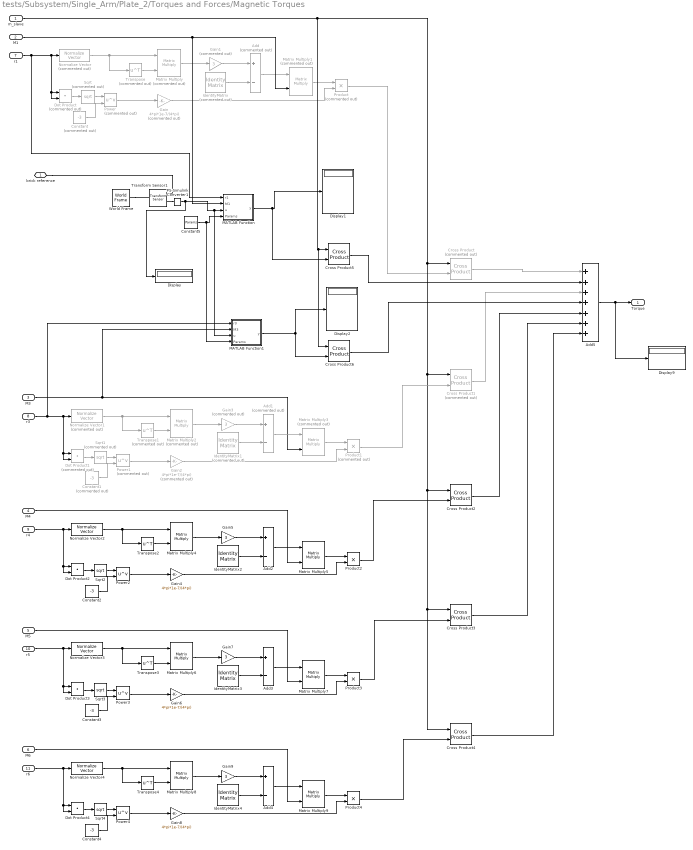
== system tests/Subsystem/Single_Arm/Plate_2/Torques and Forces/Magnetic Torques ==
  m_slave : Inport
  M1 : Inport  Port=2
  M3 : Inport  Port=3
  M4 : Inport  Port=4
  M5 : Inport  Port=5
  M6 : Inport  Port=6
  r1 : Inport  Port=7
  r3 : Inport  Port=8
  r4 : Inport  Port=9
  r5 : Inport  Port=10
  r6 : Inport  Port=11
  Add : Sum  Commented=on  Inputs=+-
  Add1 : Sum  Commented=on  Inputs=+-
  Add2 : Sum  Inputs=+-
  Add3 : Sum  Inputs=+-
  Add4 : Sum  Inputs=+-
  Add5 : Sum  Inputs=+++++++
  Constant : Constant  Commented=on  Value=-3
  Constant1 : Constant  Commented=on  Value=-3
  Constant2 : Constant  Value=-3
  Constant3 : Constant  Value=-3
  Constant4 : Constant  Value=-3
  Constant5 : Constant  Value=Params  OutDataTypeStr=Bus:slBus1
  Cross Product : matrix_library/Cross Product  Commented=on
  Cross Product1 : matrix_library/Cross Product  Commented=on
  Cross Product{2..6} (5 alike) : matrix_library/Cross Product
  Display{,1..2,9} (4 alike) : Display
  Dot Product : DotProduct  Commented=on  OutDataTypeStr=Inherit: Inherit via internal rule
  Dot Product1 : DotProduct  Commented=on  OutDataTypeStr=Inherit: Inherit via internal rule
  Dot Product2 : DotProduct  OutDataTypeStr=Inherit: Inherit via internal rule
  Dot Product3 : DotProduct  OutDataTypeStr=Inherit: Inherit via internal rule
  Dot Product4 : DotProduct  OutDataTypeStr=Inherit: Inherit via internal rule
  Gain : Gain  Commented=on  Gain=4*pi*1e-7/(4*pi)
  Gain1 : Gain  Commented=on  Gain=3
  Gain2 : Gain  Commented=on  Gain=4*pi*1e-7/(4*pi)
  Gain3 : Gain  Commented=on  Gain=3
  Gain4 : Gain  Gain=4*pi*1e-7/(4*pi)
  Gain5 : Gain  Gain=3
  Gain6 : Gain  Gain=4*pi*1e-7/(4*pi)
  Gain7 : Gain  Gain=3
  Gain8 : Gain  Gain=4*pi*1e-7/(4*pi)
  Gain9 : Gain  Gain=3
  IdentityMatrix : IdentityMatrix  Commented=on  OutputDimensions=3
  IdentityMatrix1 : IdentityMatrix  Commented=on  OutputDimensions=3
  IdentityMatrix2 : IdentityMatrix  OutputDimensions=3
  IdentityMatrix3 : IdentityMatrix  OutputDimensions=3
  IdentityMatrix4 : IdentityMatrix  OutputDimensions=3
  MATLAB Function : MATLAB Function  TreatAsAtomicUnit=on
  MATLAB Function1 : MATLAB Function  TreatAsAtomicUnit=on
  Matrix Multiply{,1..3} (4 alike) : Product  Commented=on  Multiplication=Matrix(*)
  Matrix Multiply{4..9} (6 alike) : Product  Multiplication=Matrix(*)
  Normalize Vector : vrlib/Utilities/Normalize Vector  Commented=on  maxzero=0
  Normalize Vector1 : vrlib/Utilities/Normalize Vector  Commented=on  maxzero=0
  Normalize Vector2 : vrlib/Utilities/Normalize Vector  maxzero=0
  Normalize Vector3 : vrlib/Utilities/Normalize Vector  maxzero=0
  Normalize Vector4 : vrlib/Utilities/Normalize Vector  maxzero=0
  PS-Simulink Converter1 : nesl_utility/PS-Simulink Converter  PhysicalDomain=network_engine_domain  SubClassName=ps_output  LeftPortType=input  RightPortType=output  PseudoPeriodic=off  Frequencies=[]  VectorFormat=inherit  Unit=inherit  AffineConversion=off
  Power : Math  Commented=on  Operator=pow
  Power1 : Math  Commented=on  Operator=pow
  Power2 : Math  Operator=pow
  Power3 : Math  Operator=pow
  Power4 : Math  Operator=pow
  Product : Product  Commented=on
  Product1 : Product  Commented=on
  Product2 : Product
  Product3 : Product
  Product4 : Product
  Sqrt : Sqrt  Commented=on
  Sqrt1 : Sqrt  Commented=on
  Sqrt2 : Sqrt
  Sqrt3 : Sqrt
  Sqrt4 : Sqrt
  Transform Sensor1 : sm_lib/Frames and Transforms/Transform Sensor  MeasurementFrame=World  RotationSequence=XYX  SenseAngle=off  SenseAxis=off  SenseQ=off  SenseR=on  SenseRotationSequence=off  SenseOmegaX=off  SenseOmegaY=off  SenseOmegaZ=off  SenseOmega=off  SenseQDot=off  SenseRDot=off  SenseRotationSequenceDot=off  SenseAlphaX=off  SenseAlphaY=off  SenseAlphaZ=off  SenseAlpha=off  SenseQDDot=off  SenseRDDot=off  SenseX=off  SenseY=off  SenseZ=off  SenseXYZ=off  SenseRad=off  SenseAzim=off  SenseDist=off  SenseInc=off  SenseXDot=off  SenseYDot=off  SenseZDot=off  SenseXYZDot=off  SenseRadDot=off  SenseAzimDot=off  SenseDistDot=off  SenseIncDot=off  SenseXDDot=off  SenseYDDot=off  SenseZDDot=off  SenseXYZDDot=off  SenseRadDDot=off  SenseAzimDDot=off  SenseDistDDot=off  SenseIncDDot=off
  Transpose : Math  Commented=on  Operator=transpose
  Transpose1 : Math  Commented=on  Operator=transpose
  Transpose2 : Math  Operator=transpose
  Transpose3 : Math  Operator=transpose
  Transpose4 : Math  Operator=transpose
  World Frame : sm_lib/Frames and Transforms/World Frame
  brick reference : PMIOPort  Side=Left
  Torque : Outport
  wires:
  Constant/1 -> Power/2
  Power/1 -> Gain/1
  Normalize Vector/1 -> Transpose/1, Matrix Multiply/1
  Transpose/1 -> Matrix Multiply/2
  Matrix Multiply/1 -> Gain1/1
  IdentityMatrix/1 -> Add/2
  Gain1/1 -> Add/1
  Add/1 -> Matrix Multiply1/1
  Matrix Multiply1/1 -> Product/1
  Gain/1 -> Product/2
  Product/1 -> Cross Product/2
  m_slave/1 -> Cross Product6/1, Cross Product5/1, Cross Product4/1, Cross Product3/1, Cross Product2/1, Cross Product1/1, Cross Product/1
  Dot Product/1 -> Sqrt/1
  Sqrt/1 -> Power/1
  Transpose1/1 -> Matrix Multiply2/2
  Normalize Vector1/1 -> Transpose1/1, Matrix Multiply2/1
  r3/1 -> MATLAB Function1/1(r3), Dot Product1/2, Dot Product1/1, Normalize Vector1/1
  Matrix Multiply3/1 -> Product1/1
  Matrix Multiply2/1 -> Gain3/1
  IdentityMatrix1/1 -> Add1/2
  Power1/1 -> Gain2/1
  M3/1 -> MATLAB Function1/2(M3), Matrix Multiply3/2
  Gain3/1 -> Add1/1
  Sqrt1/1 -> Power1/1
  Product1/1 -> Cross Product1/2
  Gain2/1 -> Product1/2
  Add1/1 -> Matrix Multiply3/1
  Dot Product1/1 -> Sqrt1/1
  Constant1/1 -> Power1/2
  Transpose2/1 -> Matrix Multiply4/2
  Normalize Vector2/1 -> Transpose2/1, Matrix Multiply4/1
  r4/1 -> Dot Product2/2, Dot Product2/1, Normalize Vector2/1
  Matrix Multiply5/1 -> Product2/1
  Matrix Multiply4/1 -> Gain5/1
  IdentityMatrix2/1 -> Add2/2
  Power2/1 -> Gain4/1
  M4/1 -> Matrix Multiply5/2
  Gain5/1 -> Add2/1
  Sqrt2/1 -> Power2/1
  Product2/1 -> Cross Product2/2
  Gain4/1 -> Product2/2
  Add2/1 -> Matrix Multiply5/1
  Dot Product2/1 -> Sqrt2/1
  Constant2/1 -> Power2/2
  Transpose3/1 -> Matrix Multiply6/2
  Normalize Vector3/1 -> Transpose3/1, Matrix Multiply6/1
  r5/1 -> Dot Product3/2, Dot Product3/1, Normalize Vector3/1
  Matrix Multiply7/1 -> Product3/1
  Matrix Multiply6/1 -> Gain7/1
  IdentityMatrix3/1 -> Add3/2
  Power3/1 -> Gain6/1
  M5/1 -> Matrix Multiply7/2
  Gain7/1 -> Add3/1
  Sqrt3/1 -> Power3/1
  Product3/1 -> Cross Product3/2
  Gain6/1 -> Product3/2
  Add3/1 -> Matrix Multiply7/1
  Dot Product3/1 -> Sqrt3/1
  Constant3/1 -> Power3/2
  Transpose4/1 -> Matrix Multiply8/2
  Normalize Vector4/1 -> Transpose4/1, Matrix Multiply8/1
  r6/1 -> Dot Product4/2, Dot Product4/1, Normalize Vector4/1
  Matrix Multiply9/1 -> Product4/1
  Matrix Multiply8/1 -> Gain9/1
  IdentityMatrix4/1 -> Add4/2
  Power4/1 -> Gain8/1
  M6/1 -> Matrix Multiply9/2
  Gain9/1 -> Add4/1
  Sqrt4/1 -> Power4/1
  Product4/1 -> Cross Product4/2
  Gain8/1 -> Product4/2
  Add4/1 -> Matrix Multiply9/1
  Dot Product4/1 -> Sqrt4/1
  Constant4/1 -> Power4/2
  Cross Product/1 -> Add5/1
  Cross Product1/1 -> Add5/3
  Cross Product2/1 -> Add5/5
  Cross Product3/1 -> Add5/6
  Cross Product4/1 -> Add5/7
  Add5/1 -> Display9/1, Torque/1
  MATLAB Function/1(y) -> Cross Product5/2, Display1/1
  PS-Simulink Converter1/1 -> Display/1, MATLAB Function1/3(u), MATLAB Function/3(u)
  M1/1 -> MATLAB Function/2(M1), Matrix Multiply1/2
  Constant5/1 -> MATLAB Function1/4(Params), MATLAB Function/4(Params)
  r1/1 -> MATLAB Function/1(r1), Dot Product/2, Dot Product/1, Normalize Vector/1
  Cross Product5/1 -> Add5/2
  MATLAB Function1/1(y) -> Display2/1, Cross Product6/2
  Cross Product6/1 -> Add5/4
  connections:
  World Frame/RConn1 -- Transform Sensor1/LConn1
  brick reference/RConn1 -- Transform Sensor1/RConn1
  Transform Sensor1/RConn2 -- PS-Simulink Converter1/LConn1
